simulink model "V40"  (R2017b)
settings: Solver=FixedStepAuto  StartTime=0.0  StopTime=50  FixedStep=dt  RelTol=1e-3
undefined symbols (not defined in the file): b_ref, c_bar, CG_ref_x, CG_ref_z, CL0, Clp, Clr, Cm0, Cmq, Cnp, Cnr, CX_d_ca_l, CX_d_ca_r, CX_d_ea_l, CX_d_ea_r, CX_d_r, d_ca_trim, D_CL_alpha, D_Cm_alpha, DCD_alpha, DCX_beta, dt, Earth, FW_P_RMAX_POS, FW_P_TC, FW_PR_FF, FW_PR_I, FW_PR_IMAX, FW_PR_P, FW_R_RMAX, FW_R_TC, FW_RR_FF, FW_RR_I, FW_RR_IMAX, FW_RR_P, FW_YR_FF, FW_YR_I, FW_YR_IMAX, FW_YR_P, g, h0, hgt_error_gain, hgt_gain_ff, K_L1, L1_ratio, lat0, lon0, mass0, max_climb_rate, max_sink_rate, min_sink_rate, Newton, p0, pitch0, Pitch_Kd, Pitch_Ki, pitch_sp_limit, pitch_time_constant, q0, r0 ... (+28)
libraries: simulink_extras x6, aerolibtransform2 x2, shared6dof x1, aerolibasang x1, simulink x1
(part 2 of 2)

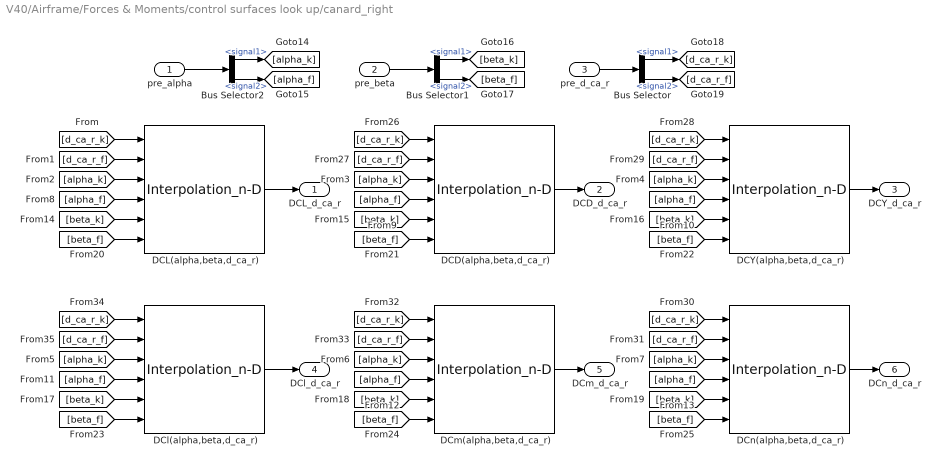
== system V40/Airframe/Forces & Moments/control surfaces look up/canard_right ==
  pre_alpha : Inport
  pre_beta : Inport  Port=2
  pre_d_ca_r : Inport  Port=3
  Bus Selector : BusSelector  OutputSignals=signal1,signal2
  Bus Selector1 : BusSelector  OutputSignals=signal1,signal2
  Bus Selector2 : BusSelector  OutputSignals=signal1,signal2
  DCD(alpha,beta,d_ca_r) : Interpolation_n-D  NumberOfTableDimensions=3  Table=CX_d_ca_r{2}  OutDataTypeStr=single
      settings: InputPortMap=u0,u1,u2,u3,u4,u5
  DCL(alpha,beta,d_ca_r) : Interpolation_n-D  NumberOfTableDimensions=3  Table=CX_d_ca_r{1}  OutDataTypeStr=single
      settings: InputPortMap=u0,u1,u2,u3,u4,u5
  DCY(alpha,beta,d_ca_r) : Interpolation_n-D  NumberOfTableDimensions=3  Table=CX_d_ca_r{4}  OutDataTypeStr=single
      settings: InputPortMap=u0,u1,u2,u3,u4,u5
  DCl(alpha,beta,d_ca_r) : Interpolation_n-D  NumberOfTableDimensions=3  Table=CX_d_ca_r{6}  OutDataTypeStr=single
      settings: InputPortMap=u0,u1,u2,u3,u4,u5
  DCm(alpha,beta,d_ca_r) : Interpolation_n-D  NumberOfTableDimensions=3  Table=CX_d_ca_r{3}  OutDataTypeStr=single
      settings: InputPortMap=u0,u1,u2,u3,u4,u5
  DCn(alpha,beta,d_ca_r) : Interpolation_n-D  NumberOfTableDimensions=3  Table=CX_d_ca_r{5}  OutDataTypeStr=single
      settings: InputPortMap=u0,u1,u2,u3,u4,u5
  DCL_d_ca_r : Outport
  DCD_d_ca_r : Outport  Port=2
  DCY_d_ca_r : Outport  Port=3
  DCl_d_ca_r : Outport  Port=4
  DCm_d_ca_r : Outport  Port=5
  DCn_d_ca_r : Outport  Port=6
  wires:
  Bus Selector1/2 -> [beta_f]  "<signal2>"
  DCY(alpha,beta,d_ca_r)/1 -> DCY_d_ca_r/1
  pre_beta/1 -> Bus Selector1/1
  Bus Selector/2 -> [d_ca_r_f]  "<signal2>"
  DCD(alpha,beta,d_ca_r)/1 -> DCD_d_ca_r/1
  DCl(alpha,beta,d_ca_r)/1 -> DCl_d_ca_r/1
  Bus Selector/1 -> [d_ca_r_k]  "<signal1>"
  Bus Selector2/1 -> [alpha_k]  "<signal1>"
  DCm(alpha,beta,d_ca_r)/1 -> DCm_d_ca_r/1
  Bus Selector2/2 -> [alpha_f]  "<signal2>"
  pre_alpha/1 -> Bus Selector2/1
  DCn(alpha,beta,d_ca_r)/1 -> DCn_d_ca_r/1
  DCL(alpha,beta,d_ca_r)/1 -> DCL_d_ca_r/1
  Bus Selector1/1 -> [beta_k]  "<signal1>"
  [d_ca_r_k] -> DCD(alpha,beta,d_ca_r)/1
  [beta_k] -> DCD(alpha,beta,d_ca_r)/5
  [d_ca_r_k] -> DCY(alpha,beta,d_ca_r)/1
  [beta_k] -> DCY(alpha,beta,d_ca_r)/5
  [alpha_k] -> DCY(alpha,beta,d_ca_r)/3
  [d_ca_r_k] -> DCn(alpha,beta,d_ca_r)/1
  [beta_k] -> DCn(alpha,beta,d_ca_r)/5
  [d_ca_r_k] -> DCm(alpha,beta,d_ca_r)/1
  [beta_k] -> DCm(alpha,beta,d_ca_r)/5
  [d_ca_r_k] -> DCL(alpha,beta,d_ca_r)/1
  [d_ca_r_f] -> DCL(alpha,beta,d_ca_r)/2
  [alpha_k] -> DCL(alpha,beta,d_ca_r)/3
  [alpha_f] -> DCL(alpha,beta,d_ca_r)/4
  [beta_k] -> DCL(alpha,beta,d_ca_r)/5
  [beta_f] -> DCL(alpha,beta,d_ca_r)/6
  [d_ca_r_f] -> DCD(alpha,beta,d_ca_r)/2
  [alpha_k] -> DCD(alpha,beta,d_ca_r)/3
  [alpha_f] -> DCD(alpha,beta,d_ca_r)/4
  [beta_f] -> DCD(alpha,beta,d_ca_r)/6
  [d_ca_r_f] -> DCY(alpha,beta,d_ca_r)/2
  [alpha_f] -> DCY(alpha,beta,d_ca_r)/4
  [beta_f] -> DCY(alpha,beta,d_ca_r)/6
  [d_ca_r_f] -> DCn(alpha,beta,d_ca_r)/2
  [alpha_k] -> DCn(alpha,beta,d_ca_r)/3
  [alpha_f] -> DCn(alpha,beta,d_ca_r)/4
  [beta_f] -> DCn(alpha,beta,d_ca_r)/6
  [d_ca_r_f] -> DCm(alpha,beta,d_ca_r)/2
  [alpha_k] -> DCm(alpha,beta,d_ca_r)/3
  [alpha_f] -> DCm(alpha,beta,d_ca_r)/4
  [beta_f] -> DCm(alpha,beta,d_ca_r)/6
  [d_ca_r_k] -> DCl(alpha,beta,d_ca_r)/1
  [d_ca_r_f] -> DCl(alpha,beta,d_ca_r)/2
  [alpha_k] -> DCl(alpha,beta,d_ca_r)/3
  [alpha_f] -> DCl(alpha,beta,d_ca_r)/4
  [beta_k] -> DCl(alpha,beta,d_ca_r)/5
  [beta_f] -> DCl(alpha,beta,d_ca_r)/6
  pre_d_ca_r/1 -> Bus Selector/1

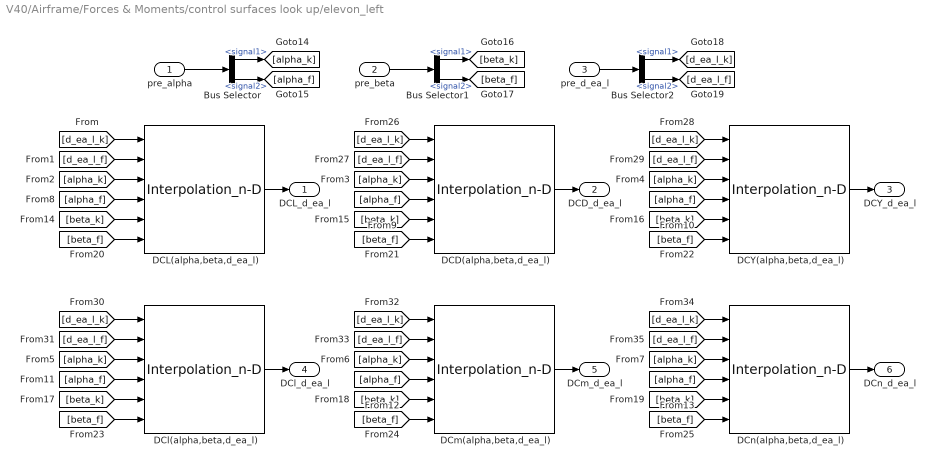
== system V40/Airframe/Forces & Moments/control surfaces look up/elevon_left  ==
  pre_alpha : Inport
  pre_beta : Inport  Port=2
  pre_d_ea_l : Inport  Port=3
  Bus Selector : BusSelector  OutputSignals=signal1,signal2
  Bus Selector1 : BusSelector  OutputSignals=signal1,signal2
  Bus Selector2 : BusSelector  OutputSignals=signal1,signal2
  DCD(alpha,beta,d_ea_l) : Interpolation_n-D  NumberOfTableDimensions=3  Table=CX_d_ea_l{2}  OutDataTypeStr=single
      settings: InputPortMap=u0,u1,u2,u3,u4,u5
  DCL(alpha,beta,d_ea_l) : Interpolation_n-D  NumberOfTableDimensions=3  Table=CX_d_ea_l{1}  OutDataTypeStr=single
      settings: InputPortMap=u0,u1,u2,u3,u4,u5
  DCY(alpha,beta,d_ea_l) : Interpolation_n-D  NumberOfTableDimensions=3  Table=CX_d_ea_l{4}  OutDataTypeStr=single
      settings: InputPortMap=u0,u1,u2,u3,u4,u5
  DCl(alpha,beta,d_ea_l) : Interpolation_n-D  NumberOfTableDimensions=3  Table=CX_d_ea_l{6}  OutDataTypeStr=single
      settings: InputPortMap=u0,u1,u2,u3,u4,u5
  DCm(alpha,beta,d_ea_l) : Interpolation_n-D  NumberOfTableDimensions=3  Table=CX_d_ea_l{3}  OutDataTypeStr=single
      settings: InputPortMap=u0,u1,u2,u3,u4,u5
  DCn(alpha,beta,d_ea_l) : Interpolation_n-D  NumberOfTableDimensions=3  Table=CX_d_ea_l{5}  OutDataTypeStr=single
      settings: InputPortMap=u0,u1,u2,u3,u4,u5
  DCL_d_ea_l : Outport
  DCD_d_ea_l : Outport  Port=2
  DCY_d_ea_l : Outport  Port=3
  DCl_d_ea_l : Outport  Port=4
  DCm_d_ea_l : Outport  Port=5
  DCn_d_ea_l : Outport  Port=6
  wires:
  Bus Selector1/2 -> [beta_f]  "<signal2>"
  DCY(alpha,beta,d_ea_l)/1 -> DCY_d_ea_l/1
  pre_beta/1 -> Bus Selector1/1
  Bus Selector2/2 -> [d_ea_l_f]  "<signal2>"
  DCD(alpha,beta,d_ea_l)/1 -> DCD_d_ea_l/1
  DCl(alpha,beta,d_ea_l)/1 -> DCl_d_ea_l/1
  Bus Selector2/1 -> [d_ea_l_k]  "<signal1>"
  Bus Selector/1 -> [alpha_k]  "<signal1>"
  DCm(alpha,beta,d_ea_l)/1 -> DCm_d_ea_l/1
  Bus Selector/2 -> [alpha_f]  "<signal2>"
  pre_alpha/1 -> Bus Selector/1
  DCn(alpha,beta,d_ea_l)/1 -> DCn_d_ea_l/1
  DCL(alpha,beta,d_ea_l)/1 -> DCL_d_ea_l/1
  Bus Selector1/1 -> [beta_k]  "<signal1>"
  [beta_k] -> DCL(alpha,beta,d_ea_l)/5
  [beta_f] -> DCL(alpha,beta,d_ea_l)/6
  [beta_k] -> DCD(alpha,beta,d_ea_l)/5
  [beta_f] -> DCD(alpha,beta,d_ea_l)/6
  [beta_k] -> DCY(alpha,beta,d_ea_l)/5
  [beta_f] -> DCY(alpha,beta,d_ea_l)/6
  [beta_k] -> DCl(alpha,beta,d_ea_l)/5
  [beta_f] -> DCl(alpha,beta,d_ea_l)/6
  [beta_k] -> DCm(alpha,beta,d_ea_l)/5
  [beta_f] -> DCm(alpha,beta,d_ea_l)/6
  [beta_k] -> DCn(alpha,beta,d_ea_l)/5
  [beta_f] -> DCn(alpha,beta,d_ea_l)/6
  [d_ea_l_k] -> DCD(alpha,beta,d_ea_l)/1
  [d_ea_l_k] -> DCY(alpha,beta,d_ea_l)/1
  [d_ea_l_k] -> DCn(alpha,beta,d_ea_l)/1
  [alpha_k] -> DCn(alpha,beta,d_ea_l)/3
  [d_ea_l_k] -> DCm(alpha,beta,d_ea_l)/1
  [alpha_k] -> DCm(alpha,beta,d_ea_l)/3
  [d_ea_l_k] -> DCl(alpha,beta,d_ea_l)/1
  [alpha_k] -> DCl(alpha,beta,d_ea_l)/3
  [d_ea_l_k] -> DCL(alpha,beta,d_ea_l)/1
  [d_ea_l_f] -> DCL(alpha,beta,d_ea_l)/2
  [alpha_k] -> DCL(alpha,beta,d_ea_l)/3
  [alpha_f] -> DCL(alpha,beta,d_ea_l)/4
  [d_ea_l_f] -> DCD(alpha,beta,d_ea_l)/2
  [alpha_k] -> DCD(alpha,beta,d_ea_l)/3
  [alpha_f] -> DCD(alpha,beta,d_ea_l)/4
  [d_ea_l_f] -> DCY(alpha,beta,d_ea_l)/2
  [alpha_k] -> DCY(alpha,beta,d_ea_l)/3
  [alpha_f] -> DCY(alpha,beta,d_ea_l)/4
  [d_ea_l_f] -> DCn(alpha,beta,d_ea_l)/2
  [alpha_f] -> DCn(alpha,beta,d_ea_l)/4
  [d_ea_l_f] -> DCm(alpha,beta,d_ea_l)/2
  [alpha_f] -> DCm(alpha,beta,d_ea_l)/4
  [d_ea_l_f] -> DCl(alpha,beta,d_ea_l)/2
  [alpha_f] -> DCl(alpha,beta,d_ea_l)/4
  pre_d_ea_l/1 -> Bus Selector2/1

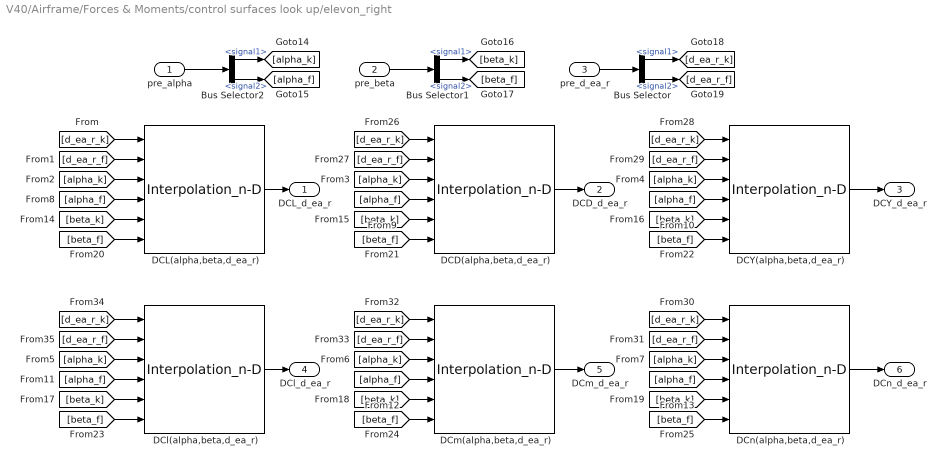
== system V40/Airframe/Forces & Moments/control surfaces look up/elevon_right  ==
  pre_alpha : Inport
  pre_beta : Inport  Port=2
  pre_d_ea_r : Inport  Port=3
  Bus Selector : BusSelector  OutputSignals=signal1,signal2
  Bus Selector1 : BusSelector  OutputSignals=signal1,signal2
  Bus Selector2 : BusSelector  OutputSignals=signal1,signal2
  DCD(alpha,beta,d_ea_r) : Interpolation_n-D  NumberOfTableDimensions=3  Table=CX_d_ea_r{2}  OutDataTypeStr=single
      settings: InputPortMap=u0,u1,u2,u3,u4,u5
  DCL(alpha,beta,d_ea_r) : Interpolation_n-D  NumberOfTableDimensions=3  Table=CX_d_ea_r{1}  OutDataTypeStr=single
      settings: InputPortMap=u0,u1,u2,u3,u4,u5
  DCY(alpha,beta,d_ea_r) : Interpolation_n-D  NumberOfTableDimensions=3  Table=CX_d_ea_r{4}  OutDataTypeStr=single
      settings: InputPortMap=u0,u1,u2,u3,u4,u5
  DCl(alpha,beta,d_ea_r) : Interpolation_n-D  NumberOfTableDimensions=3  Table=CX_d_ea_r{6}  OutDataTypeStr=single
      settings: InputPortMap=u0,u1,u2,u3,u4,u5
  DCm(alpha,beta,d_ea_r) : Interpolation_n-D  NumberOfTableDimensions=3  Table=CX_d_ea_r{3}  OutDataTypeStr=single
      settings: InputPortMap=u0,u1,u2,u3,u4,u5
  DCn(alpha,beta,d_ea_r) : Interpolation_n-D  NumberOfTableDimensions=3  Table=CX_d_ea_r{5}  OutDataTypeStr=single
      settings: InputPortMap=u0,u1,u2,u3,u4,u5
  DCL_d_ea_r : Outport
  DCD_d_ea_r : Outport  Port=2
  DCY_d_ea_r : Outport  Port=3
  DCl_d_ea_r : Outport  Port=4
  DCm_d_ea_r : Outport  Port=5
  DCn_d_ea_r : Outport  Port=6
  wires:
  Bus Selector1/2 -> [beta_f]  "<signal2>"
  DCY(alpha,beta,d_ea_r)/1 -> DCY_d_ea_r/1
  pre_beta/1 -> Bus Selector1/1
  Bus Selector/2 -> [d_ea_r_f]  "<signal2>"
  DCD(alpha,beta,d_ea_r)/1 -> DCD_d_ea_r/1
  DCl(alpha,beta,d_ea_r)/1 -> DCl_d_ea_r/1
  Bus Selector/1 -> [d_ea_r_k]  "<signal1>"
  Bus Selector2/1 -> [alpha_k]  "<signal1>"
  DCm(alpha,beta,d_ea_r)/1 -> DCm_d_ea_r/1
  Bus Selector2/2 -> [alpha_f]  "<signal2>"
  pre_alpha/1 -> Bus Selector2/1
  DCn(alpha,beta,d_ea_r)/1 -> DCn_d_ea_r/1
  DCL(alpha,beta,d_ea_r)/1 -> DCL_d_ea_r/1
  Bus Selector1/1 -> [beta_k]  "<signal1>"
  [beta_k] -> DCL(alpha,beta,d_ea_r)/5
  [beta_f] -> DCL(alpha,beta,d_ea_r)/6
  [beta_k] -> DCD(alpha,beta,d_ea_r)/5
  [beta_f] -> DCD(alpha,beta,d_ea_r)/6
  [beta_k] -> DCY(alpha,beta,d_ea_r)/5
  [beta_f] -> DCY(alpha,beta,d_ea_r)/6
  [beta_k] -> DCl(alpha,beta,d_ea_r)/5
  [beta_f] -> DCl(alpha,beta,d_ea_r)/6
  [beta_k] -> DCm(alpha,beta,d_ea_r)/5
  [beta_f] -> DCm(alpha,beta,d_ea_r)/6
  [beta_k] -> DCn(alpha,beta,d_ea_r)/5
  [beta_f] -> DCn(alpha,beta,d_ea_r)/6
  [d_ea_r_k] -> DCD(alpha,beta,d_ea_r)/1
  [d_ea_r_k] -> DCY(alpha,beta,d_ea_r)/1
  [d_ea_r_k] -> DCn(alpha,beta,d_ea_r)/1
  [d_ea_r_k] -> DCm(alpha,beta,d_ea_r)/1
  [d_ea_r_k] -> DCL(alpha,beta,d_ea_r)/1
  [d_ea_r_f] -> DCL(alpha,beta,d_ea_r)/2
  [alpha_k] -> DCL(alpha,beta,d_ea_r)/3
  [alpha_f] -> DCL(alpha,beta,d_ea_r)/4
  [d_ea_r_f] -> DCD(alpha,beta,d_ea_r)/2
  [alpha_k] -> DCD(alpha,beta,d_ea_r)/3
  [alpha_f] -> DCD(alpha,beta,d_ea_r)/4
  [d_ea_r_f] -> DCY(alpha,beta,d_ea_r)/2
  [alpha_k] -> DCY(alpha,beta,d_ea_r)/3
  [alpha_f] -> DCY(alpha,beta,d_ea_r)/4
  [d_ea_r_f] -> DCn(alpha,beta,d_ea_r)/2
  [alpha_k] -> DCn(alpha,beta,d_ea_r)/3
  [alpha_f] -> DCn(alpha,beta,d_ea_r)/4
  [d_ea_r_f] -> DCm(alpha,beta,d_ea_r)/2
  [alpha_k] -> DCm(alpha,beta,d_ea_r)/3
  [alpha_f] -> DCm(alpha,beta,d_ea_r)/4
  [d_ea_r_k] -> DCl(alpha,beta,d_ea_r)/1
  [d_ea_r_f] -> DCl(alpha,beta,d_ea_r)/2
  [alpha_k] -> DCl(alpha,beta,d_ea_r)/3
  [alpha_f] -> DCl(alpha,beta,d_ea_r)/4
  pre_d_ea_r/1 -> Bus Selector/1

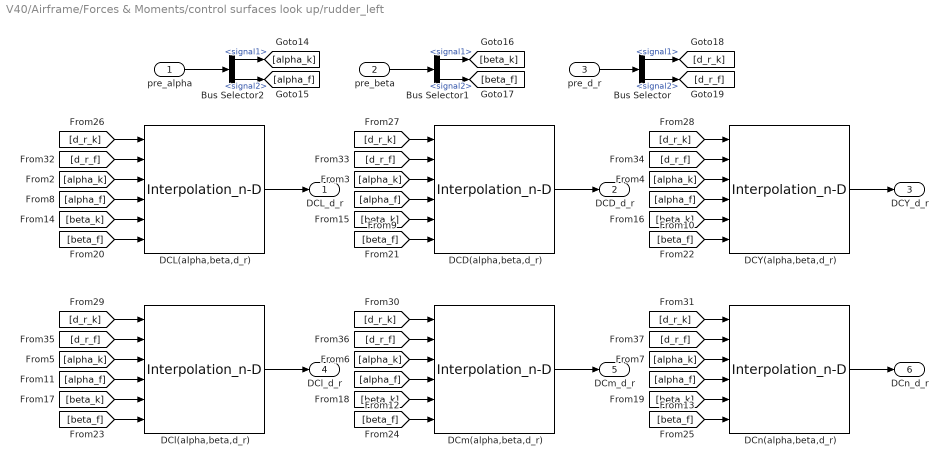
== system V40/Airframe/Forces & Moments/control surfaces look up/rudder_left ==
  pre_alpha : Inport
  pre_beta : Inport  Port=2
  pre_d_r : Inport  Port=3
  Bus Selector : BusSelector  OutputSignals=signal1,signal2
  Bus Selector1 : BusSelector  OutputSignals=signal1,signal2
  Bus Selector2 : BusSelector  OutputSignals=signal1,signal2
  DCD(alpha,beta,d_r) : Interpolation_n-D  NumberOfTableDimensions=3  Table=CX_d_r{2}  OutDataTypeStr=single
      settings: InputPortMap=u0,u1,u2,u3,u4,u5
  DCL(alpha,beta,d_r) : Interpolation_n-D  NumberOfTableDimensions=3  Table=CX_d_r{1}  OutDataTypeStr=single
      settings: InputPortMap=u0,u1,u2,u3,u4,u5
  DCY(alpha,beta,d_r) : Interpolation_n-D  NumberOfTableDimensions=3  Table=CX_d_r{4}  OutDataTypeStr=single
      settings: InputPortMap=u0,u1,u2,u3,u4,u5
  DCl(alpha,beta,d_r) : Interpolation_n-D  NumberOfTableDimensions=3  Table=CX_d_r{6}  OutDataTypeStr=single
      settings: InputPortMap=u0,u1,u2,u3,u4,u5
  DCm(alpha,beta,d_r) : Interpolation_n-D  NumberOfTableDimensions=3  Table=CX_d_r{3}  OutDataTypeStr=single
      settings: InputPortMap=u0,u1,u2,u3,u4,u5
  DCn(alpha,beta,d_r) : Interpolation_n-D  NumberOfTableDimensions=3  Table=CX_d_r{5}  OutDataTypeStr=single
      settings: InputPortMap=u0,u1,u2,u3,u4,u5
  DCL_d_r : Outport
  DCD_d_r : Outport  Port=2
  DCY_d_r : Outport  Port=3
  DCl_d_r : Outport  Port=4
  DCm_d_r : Outport  Port=5
  DCn_d_r : Outport  Port=6
  wires:
  Bus Selector1/2 -> [beta_f]  "<signal2>"
  DCY(alpha,beta,d_r)/1 -> DCY_d_r/1
  pre_beta/1 -> Bus Selector1/1
  Bus Selector/2 -> [d_r_f]  "<signal2>"
  DCD(alpha,beta,d_r)/1 -> DCD_d_r/1
  DCl(alpha,beta,d_r)/1 -> DCl_d_r/1
  Bus Selector/1 -> [d_r_k]  "<signal1>"
  Bus Selector2/1 -> [alpha_k]  "<signal1>"
  DCm(alpha,beta,d_r)/1 -> DCm_d_r/1
  Bus Selector2/2 -> [alpha_f]  "<signal2>"
  pre_alpha/1 -> Bus Selector2/1
  DCn(alpha,beta,d_r)/1 -> DCn_d_r/1
  DCL(alpha,beta,d_r)/1 -> DCL_d_r/1
  Bus Selector1/1 -> [beta_k]  "<signal1>"
  [d_r_k] -> DCD(alpha,beta,d_r)/1
  [beta_k] -> DCD(alpha,beta,d_r)/5
  [d_r_k] -> DCY(alpha,beta,d_r)/1
  [beta_k] -> DCY(alpha,beta,d_r)/5
  [alpha_k] -> DCY(alpha,beta,d_r)/3
  [d_r_k] -> DCn(alpha,beta,d_r)/1
  [beta_k] -> DCn(alpha,beta,d_r)/5
  [d_r_k] -> DCm(alpha,beta,d_r)/1
  [beta_k] -> DCm(alpha,beta,d_r)/5
  [d_r_k] -> DCL(alpha,beta,d_r)/1
  [d_r_f] -> DCL(alpha,beta,d_r)/2
  [alpha_k] -> DCL(alpha,beta,d_r)/3
  [alpha_f] -> DCL(alpha,beta,d_r)/4
  [beta_k] -> DCL(alpha,beta,d_r)/5
  [beta_f] -> DCL(alpha,beta,d_r)/6
  [d_r_f] -> DCD(alpha,beta,d_r)/2
  [alpha_k] -> DCD(alpha,beta,d_r)/3
  [alpha_f] -> DCD(alpha,beta,d_r)/4
  [beta_f] -> DCD(alpha,beta,d_r)/6
  [d_r_f] -> DCY(alpha,beta,d_r)/2
  [alpha_f] -> DCY(alpha,beta,d_r)/4
  [beta_f] -> DCY(alpha,beta,d_r)/6
  [d_r_f] -> DCn(alpha,beta,d_r)/2
  [alpha_k] -> DCn(alpha,beta,d_r)/3
  [alpha_f] -> DCn(alpha,beta,d_r)/4
  [beta_f] -> DCn(alpha,beta,d_r)/6
  [d_r_f] -> DCm(alpha,beta,d_r)/2
  [alpha_k] -> DCm(alpha,beta,d_r)/3
  [alpha_f] -> DCm(alpha,beta,d_r)/4
  [beta_f] -> DCm(alpha,beta,d_r)/6
  [d_r_k] -> DCl(alpha,beta,d_r)/1
  [d_r_f] -> DCl(alpha,beta,d_r)/2
  [alpha_k] -> DCl(alpha,beta,d_r)/3
  [alpha_f] -> DCl(alpha,beta,d_r)/4
  [beta_k] -> DCl(alpha,beta,d_r)/5
  [beta_f] -> DCl(alpha,beta,d_r)/6
  pre_d_r/1 -> Bus Selector/1

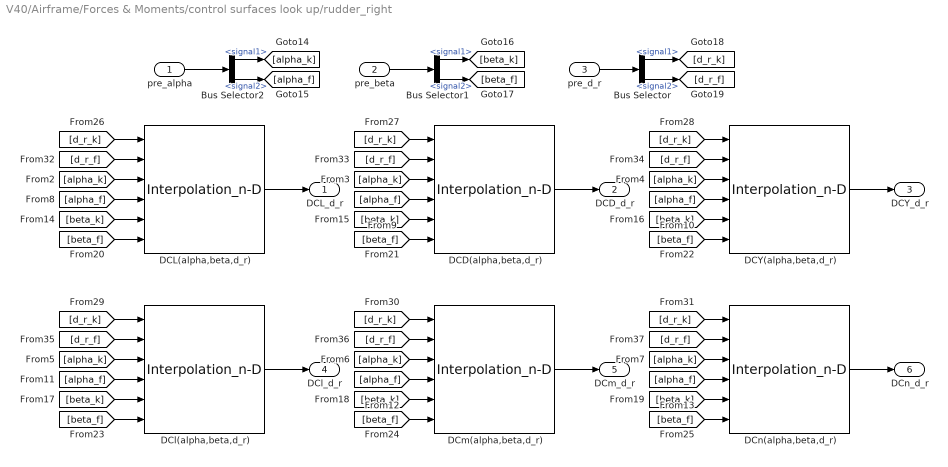
== system V40/Airframe/Forces & Moments/control surfaces look up/rudder_right ==
  pre_alpha : Inport
  pre_beta : Inport  Port=2
  pre_d_r : Inport  Port=3
  Bus Selector : BusSelector  OutputSignals=signal1,signal2
  Bus Selector1 : BusSelector  OutputSignals=signal1,signal2
  Bus Selector2 : BusSelector  OutputSignals=signal1,signal2
  DCD(alpha,beta,d_r) : Interpolation_n-D  NumberOfTableDimensions=3  Table=CX_d_r{2}  OutDataTypeStr=single
      settings: InputPortMap=u0,u1,u2,u3,u4,u5
  DCL(alpha,beta,d_r) : Interpolation_n-D  NumberOfTableDimensions=3  Table=CX_d_r{1}  OutDataTypeStr=single
      settings: InputPortMap=u0,u1,u2,u3,u4,u5
  DCY(alpha,beta,d_r) : Interpolation_n-D  NumberOfTableDimensions=3  Table=CX_d_r{4}  OutDataTypeStr=single
      settings: InputPortMap=u0,u1,u2,u3,u4,u5
  DCl(alpha,beta,d_r) : Interpolation_n-D  NumberOfTableDimensions=3  Table=CX_d_r{6}  OutDataTypeStr=single
      settings: InputPortMap=u0,u1,u2,u3,u4,u5
  DCm(alpha,beta,d_r) : Interpolation_n-D  NumberOfTableDimensions=3  Table=CX_d_r{3}  OutDataTypeStr=single
      settings: InputPortMap=u0,u1,u2,u3,u4,u5
  DCn(alpha,beta,d_r) : Interpolation_n-D  NumberOfTableDimensions=3  Table=CX_d_r{5}  OutDataTypeStr=single
      settings: InputPortMap=u0,u1,u2,u3,u4,u5
  DCL_d_r : Outport
  DCD_d_r : Outport  Port=2
  DCY_d_r : Outport  Port=3
  DCl_d_r : Outport  Port=4
  DCm_d_r : Outport  Port=5
  DCn_d_r : Outport  Port=6
  wires:
  Bus Selector1/2 -> [beta_f]  "<signal2>"
  DCY(alpha,beta,d_r)/1 -> DCY_d_r/1
  pre_beta/1 -> Bus Selector1/1
  Bus Selector/2 -> [d_r_f]  "<signal2>"
  DCD(alpha,beta,d_r)/1 -> DCD_d_r/1
  DCl(alpha,beta,d_r)/1 -> DCl_d_r/1
  Bus Selector/1 -> [d_r_k]  "<signal1>"
  Bus Selector2/1 -> [alpha_k]  "<signal1>"
  DCm(alpha,beta,d_r)/1 -> DCm_d_r/1
  Bus Selector2/2 -> [alpha_f]  "<signal2>"
  pre_alpha/1 -> Bus Selector2/1
  DCn(alpha,beta,d_r)/1 -> DCn_d_r/1
  DCL(alpha,beta,d_r)/1 -> DCL_d_r/1
  Bus Selector1/1 -> [beta_k]  "<signal1>"
  [d_r_k] -> DCD(alpha,beta,d_r)/1
  [beta_k] -> DCD(alpha,beta,d_r)/5
  [d_r_k] -> DCY(alpha,beta,d_r)/1
  [beta_k] -> DCY(alpha,beta,d_r)/5
  [alpha_k] -> DCY(alpha,beta,d_r)/3
  [d_r_k] -> DCn(alpha,beta,d_r)/1
  [beta_k] -> DCn(alpha,beta,d_r)/5
  [d_r_k] -> DCm(alpha,beta,d_r)/1
  [beta_k] -> DCm(alpha,beta,d_r)/5
  [d_r_k] -> DCL(alpha,beta,d_r)/1
  [d_r_f] -> DCL(alpha,beta,d_r)/2
  [alpha_k] -> DCL(alpha,beta,d_r)/3
  [alpha_f] -> DCL(alpha,beta,d_r)/4
  [beta_k] -> DCL(alpha,beta,d_r)/5
  [beta_f] -> DCL(alpha,beta,d_r)/6
  [d_r_f] -> DCD(alpha,beta,d_r)/2
  [alpha_k] -> DCD(alpha,beta,d_r)/3
  [alpha_f] -> DCD(alpha,beta,d_r)/4
  [beta_f] -> DCD(alpha,beta,d_r)/6
  [d_r_f] -> DCY(alpha,beta,d_r)/2
  [alpha_f] -> DCY(alpha,beta,d_r)/4
  [beta_f] -> DCY(alpha,beta,d_r)/6
  [d_r_f] -> DCn(alpha,beta,d_r)/2
  [alpha_k] -> DCn(alpha,beta,d_r)/3
  [alpha_f] -> DCn(alpha,beta,d_r)/4
  [beta_f] -> DCn(alpha,beta,d_r)/6
  [d_r_f] -> DCm(alpha,beta,d_r)/2
  [alpha_k] -> DCm(alpha,beta,d_r)/3
  [alpha_f] -> DCm(alpha,beta,d_r)/4
  [beta_f] -> DCm(alpha,beta,d_r)/6
  [d_r_k] -> DCl(alpha,beta,d_r)/1
  [d_r_f] -> DCl(alpha,beta,d_r)/2
  [alpha_k] -> DCl(alpha,beta,d_r)/3
  [alpha_f] -> DCl(alpha,beta,d_r)/4
  [beta_k] -> DCl(alpha,beta,d_r)/5
  [beta_f] -> DCl(alpha,beta,d_r)/6
  pre_d_r/1 -> Bus Selector/1

== system V40/Airframe/Forces & Moments/summation/coef computation ==
  In : Inport
  Add1 : Sum  Inputs=+++++++++
  Demux : Demux  Outputs=9
  Out : Outport
  wires:
  In/1 -> Demux/1
  Add1/1 -> Out/1
  Demux/1 -> Add1/1
  Demux/9 -> Add1/9
  Demux/8 -> Add1/8
  Demux/7 -> Add1/7
  Demux/6 -> Add1/6
  Demux/5 -> Add1/5
  Demux/4 -> Add1/4
  Demux/2 -> Add1/2
  Demux/3 -> Add1/3

== system V40/Airframe/Forces & Moments/summation/coef computation1 ==
  In : Inport
  Add1 : Sum  Inputs=++++++++
  Demux : Demux  Outputs=8
  Out : Outport
  wires:
  In/1 -> Demux/1
  Add1/1 -> Out/1
  Demux/1 -> Add1/1
  Demux/2 -> Add1/2
  Demux/3 -> Add1/3
  Demux/4 -> Add1/4
  Demux/5 -> Add1/5
  Demux/6 -> Add1/6
  Demux/7 -> Add1/7
  Demux/8 -> Add1/8

== system V40/Airframe/Forces & Moments/summation/coef computation2 ==
  In : Inport
  Add1 : Sum  Inputs=+++++++
  Demux : Demux  Outputs=7
  Out : Outport
  wires:
  In/1 -> Demux/1
  Add1/1 -> Out/1
  Demux/1 -> Add1/1
  Demux/2 -> Add1/2
  Demux/3 -> Add1/3
  Demux/4 -> Add1/4
  Demux/5 -> Add1/5
  Demux/6 -> Add1/6
  Demux/7 -> Add1/7

== system V40/Airframe/Forces & Moments/summation/coef computation3 ==
  In : Inport
  Add1 : Sum  Inputs=++++++++
  Demux : Demux  Outputs=8
  Out : Outport
  wires:
  In/1 -> Demux/1
  Add1/1 -> Out/1
  Demux/7 -> Add1/7
  Demux/1 -> Add1/1
  Demux/2 -> Add1/2
  Demux/3 -> Add1/3
  Demux/4 -> Add1/4
  Demux/5 -> Add1/5
  Demux/6 -> Add1/6
  Demux/8 -> Add1/8

== system V40/Airframe/Forces & Moments/summation/coef computation4 ==
  In : Inport
  Add1 : Sum  Inputs=++++++++++
  Demux : Demux  Outputs=10
  Out : Outport
  wires:
  Add1/1 -> Out/1
  In/1 -> Demux/1
  Demux/1 -> Add1/1
  Demux/2 -> Add1/2
  Demux/3 -> Add1/3
  Demux/4 -> Add1/4
  Demux/5 -> Add1/5
  Demux/6 -> Add1/6
  Demux/7 -> Add1/7
  Demux/8 -> Add1/8
  Demux/9 -> Add1/9
  Demux/10 -> Add1/10

== system V40/Airframe/Forces & Moments/summation/coef computation5 ==
  In : Inport
  Add1 : Sum  Inputs=++++++++
  Demux : Demux  Outputs=8
  Out : Outport
  wires:
  Add1/1 -> Out/1
  In/1 -> Demux/1
  Demux/1 -> Add1/1
  Demux/2 -> Add1/2
  Demux/3 -> Add1/3
  Demux/4 -> Add1/4
  Demux/5 -> Add1/5
  Demux/6 -> Add1/6
  Demux/7 -> Add1/7
  Demux/8 -> Add1/8

== system V40/FLY_CTRL_SYS/ATT_CTRL(PID)/U_SURF/pitch_rate_ctrl ==
  pitch_rate_sp : Inport
  pitch_rate_est : Inport  Port=2
  FW_PR_FF : Gain  Gain=FW_PR_FF
  FW_PR_I : Gain  Gain=FW_PR_I
  FW_PR_P : Gain  Gain=FW_PR_P
  Integrator Limited1 : Integrator  LimitOutput=on  UpperSaturationLimit=FW_PR_IMAX  LowerSaturationLimit=-FW_PR_IMAX
  Saturation3 : Saturate  UpperLimit=1  LowerLimit=-1
  Sum4 : Sum  Inputs=|+-
  Sum5 : Sum  Inputs=+++
  u_pitch : Outport
  wires:
  Saturation3/1 -> u_pitch/1
  FW_PR_FF/1 -> Sum5/1
  pitch_rate_est/1 -> Sum4/2
  Sum5/1 -> Saturation3/1
  pitch_rate_sp/1 -> Sum4/1, FW_PR_FF/1
  FW_PR_P/1 -> Sum5/2
  Sum4/1 -> FW_PR_I/1, FW_PR_P/1
  Integrator Limited1/1 -> Sum5/3
  FW_PR_I/1 -> Integrator Limited1/1

== system V40/FLY_CTRL_SYS/ATT_CTRL(PID)/U_SURF/roll_rate_ctrl ==
  roll_rate_sp : Inport
  roll_rate_est : Inport  Port=2
  FW_RR_FF : Gain  Gain=FW_RR_FF
  FW_RR_I : Gain  Gain=FW_RR_I
  FW_RR_P : Gain  Gain=FW_RR_P
  Integrator Limited1 : Integrator  LimitOutput=on  UpperSaturationLimit=FW_RR_IMAX  LowerSaturationLimit=-FW_RR_IMAX
  Saturation3 : Saturate  UpperLimit=1  LowerLimit=-1
  Sum4 : Sum  Inputs=|+-
  Sum5 : Sum  Inputs=+++
  u_roll : Outport
  wires:
  Saturation3/1 -> u_roll/1
  FW_RR_FF/1 -> Sum5/1
  roll_rate_est/1 -> Sum4/2
  Sum5/1 -> Saturation3/1
  roll_rate_sp/1 -> Sum4/1, FW_RR_FF/1
  FW_RR_P/1 -> Sum5/2
  Sum4/1 -> FW_RR_P/1, FW_RR_I/1
  Integrator Limited1/1 -> Sum5/3
  FW_RR_I/1 -> Integrator Limited1/1

== system V40/FLY_CTRL_SYS/ATT_CTRL(PID)/U_SURF/yaw_rate_ctrl ==
  yaw_rate_sp : Inport
  yaw_rate_est : Inport  Port=2
  FW_YR_FF : Gain  Gain=FW_YR_FF
  FW_YR_I : Gain  Gain=FW_YR_I
  FW_YR_P : Gain  Gain=FW_YR_P
  Integrator Limited1 : Integrator  LimitOutput=on  UpperSaturationLimit=FW_YR_IMAX  LowerSaturationLimit=-FW_YR_IMAX
  Saturation3 : Saturate  UpperLimit=1  LowerLimit=-1
  Sum4 : Sum  Inputs=|+-
  Sum5 : Sum  Inputs=+++
  u_yaw : Outport
  wires:
  Saturation3/1 -> u_yaw/1
  FW_YR_FF/1 -> Sum5/1
  yaw_rate_est/1 -> Sum4/2
  Sum5/1 -> Saturation3/1
  yaw_rate_sp/1 -> Sum4/1, FW_YR_FF/1
  FW_YR_P/1 -> Sum5/2
  Sum4/1 -> FW_YR_I/1, FW_YR_P/1
  Integrator Limited1/1 -> Sum5/3
  FW_YR_I/1 -> Integrator Limited1/1

== system V40/FLY_CTRL_SYS/Guidance_Law/L1/Switch Case Action Subsystem ==
  vec_A2plane_UNIT : Inport
  ground_v_2d : Inport  Port=2
  Action Port : ActionPort  ActionType=case
  Demux : Demux  Outputs=2
  Dot Product1 : DotProduct  InputSameDT=on  OutDataTypeStr=Inherit: Inherit via internal rule
  Gain : Gain  Gain=-1
  MATLAB Function5 : MATLAB Function  TreatAsAtomicUnit=on
  Trigonometric Function : Trigonometry  Operator=atan2
  Trigonometric Function1 : Trigonometry  Operator=atan2
  eta : Outport
  nav_bearing : Outport  Port=2
  wires:
  vec_A2plane_UNIT/1 -> Gain/1
  ground_v_2d/1 -> Dot Product1/1, MATLAB Function5/1(vec1)
  Gain/1 -> Demux/1, Dot Product1/2, MATLAB Function5/2(vec2)
  MATLAB Function5/1(vec_mol) -> Trigonometric Function/1
  Dot Product1/1 -> Trigonometric Function/2
  Trigonometric Function/1 -> eta/1
  Demux/2 -> Trigonometric Function1/1
  Demux/1 -> Trigonometric Function1/2
  Trigonometric Function1/1 -> nav_bearing/1

== system V40/FLY_CTRL_SYS/Guidance_Law/L1/Switch Case Action Subsystem1 ==
  vec_B2plane_UNIT : Inport
  ground_v_2d : Inport  Port=2
  Action Port : ActionPort  ActionType=case
  Demux : Demux  Outputs=2
  Dot Product1 : DotProduct  InputSameDT=on  OutDataTypeStr=Inherit: Inherit via internal rule
  Gain : Gain  Gain=-1
  MATLAB Function5 : MATLAB Function  TreatAsAtomicUnit=on
  Trigonometric Function : Trigonometry  Operator=atan2
  Trigonometric Function1 : Trigonometry  Operator=atan2
  eta : Outport
  nav_bearing : Outport  Port=2
  wires:
  vec_B2plane_UNIT/1 -> Gain/1
  Gain/1 -> Demux/1, Dot Product1/2, MATLAB Function5/2(vec2)
  Trigonometric Function1/1 -> nav_bearing/1
  Demux/2 -> Trigonometric Function1/1
  Demux/1 -> Trigonometric Function1/2
  Dot Product1/1 -> Trigonometric Function/2
  Trigonometric Function/1 -> eta/1
  MATLAB Function5/1(vec_mol) -> Trigonometric Function/1
  ground_v_2d/1 -> MATLAB Function5/1(vec1), Dot Product1/1

== system V40/FLY_CTRL_SYS/Guidance_Law/L1/Switch Case Action Subsystem2 ==
  vec_AB_UNIT : Inport
  vec_A2plane : Inport  Port=2
  ground_v_2d : Inport  Port=3
  L1_distance : Inport  Port=4
  Action Port : ActionPort  ActionType=case
  Add : Sum
  Add1 : Sum
  Constant : Constant  Value=0.1
  Demux : Demux  Outputs=2
  Divide : Product  Inputs=*/
  Dot Product1 : DotProduct  InputSameDT=on  OutDataTypeStr=Inherit: Inherit via internal rule
  MATLAB Function1 : MATLAB Function  TreatAsAtomicUnit=on
  MATLAB Function5 : MATLAB Function  TreatAsAtomicUnit=on
  Saturation : Saturate  UpperLimit=0.7071  LowerLimit=-0.7071
  Switch : Switch  Criteria=u2 > Threshold  Threshold=0.1
  Trigonometric Function : Trigonometry  Operator=atan2
  Trigonometric Function1 : Trigonometry  Operator=asin
  Trigonometric Function2 : Trigonometry  Operator=atan2
  eta : Outport
  nav_bearing : Outport  Port=2
  wires:
  vec_AB_UNIT/1 -> Demux/1, MATLAB Function1/2(vec2), Dot Product1/2, MATLAB Function5/2(vec2)
  ground_v_2d/1 -> MATLAB Function5/1(vec1), Dot Product1/1
  MATLAB Function5/1(vec_mol) -> Trigonometric Function/1
  Dot Product1/1 -> Trigonometric Function/2
  Trigonometric Function/1 -> Add/1  "eta2"
  vec_A2plane/1 -> MATLAB Function1/1(vec1)
  MATLAB Function1/1(vec_mol) -> Divide/1
  L1_distance/1 -> Switch/2, Switch/1
  Constant/1 -> Switch/3
  Switch/1 -> Divide/2
  Divide/1 -> Saturation/1
  Saturation/1 -> Trigonometric Function1/1
  Trigonometric Function1/1 -> Add/2, Add1/1  "eta1"
  Add/1 -> eta/1
  Demux/1 -> Trigonometric Function2/2
  Demux/2 -> Trigonometric Function2/1
  Trigonometric Function2/1 -> Add1/2
  Add1/1 -> nav_bearing/1

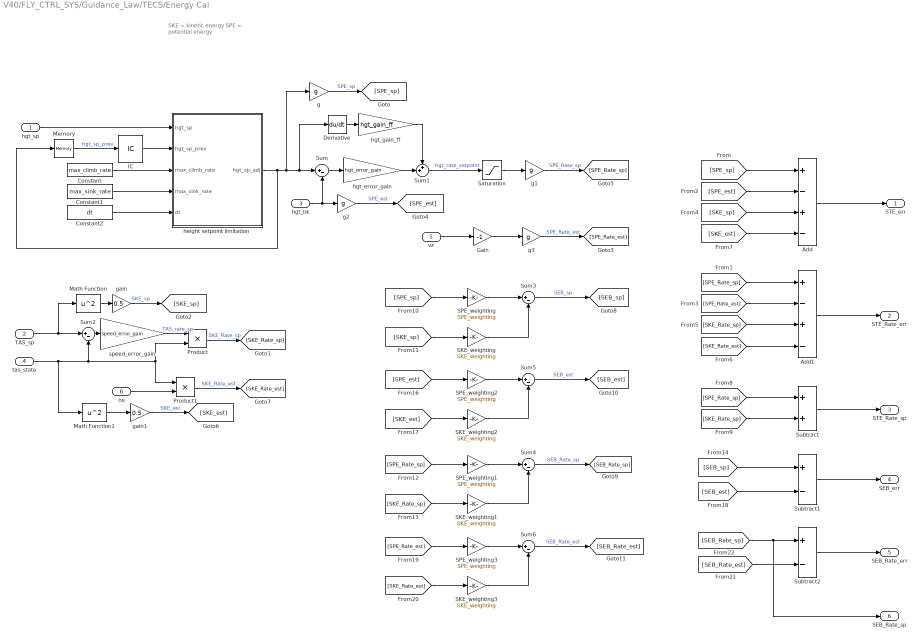
== system V40/FLY_CTRL_SYS/Guidance_Law/TECS/Energy Cal ==
  note: SKE = kinetic energy
      | SPE = potential energy
  hgt_sp : Inport
  TAS_sp : Inport  Port=2
  hgt_bk : Inport  Port=3
  tas_state : Inport  Port=4
  vz : Inport  Port=5
  nx : Inport  Port=6
  Add : Sum  Inputs=+-+-
  Add1 : Sum  Inputs=+-+-
  Constant : Constant  Value=max_climb_rate
  Constant1 : Constant  Value=max_sink_rate
  Constant2 : Constant  Value=dt
  Derivative : Derivative
  Gain : Gain  Gain=-1
  IC : InitialCondition  Value=-z0
  Math Function : Math  Operator=square  SaturateOnIntegerOverflow=on
  Math Function1 : Math  Operator=square  SaturateOnIntegerOverflow=on
  Memory : Memory
  Product : Product
  Product1 : Product
  SKE_weighting{,1..3} (4 alike) : Gain  Gain=SKE_weighting
  SPE_weighting{,1..3} (4 alike) : Gain  Gain=SPE_weighting
  Saturation : Saturate  UpperLimit=max_climb_rate  LowerLimit=-min_sink_rate
  Subtract : Sum
  Subtract1 : Sum  Inputs=+-
  Subtract2 : Sum  Inputs=+-
  Sum{,2..6} (6 alike) : Sum  Inputs=|+-
  Sum1 : Sum  Inputs=++|
  g{,1..3} (4 alike) : Gain  Gain=g
  gain : Gain  Gain=0.5
  gain1 : Gain  Gain=0.5
  height setpoint limitation : MATLAB Function  TreatAsAtomicUnit=on
  hgt_error_gain : Gain  Gain=hgt_error_gain
  hgt_gain_ff : Gain  Gain=hgt_gain_ff
  speed_error_gain : Gain  Gain=speed_error_gain
  STE_err : Outport
  STE_Rate_err : Outport  Port=2
  STE_Rate_sp : Outport  Port=3
  SEB_err : Outport  Port=4
  SEB_Rate_err : Outport  Port=5
  SEB_Rate_sp : Outport  Port=6
  wires:
  [SKE_est] -> Add/4
  vz/1 -> Gain/1
  Add1/1 -> STE_Rate_err/1
  hgt_error_gain/1 -> Sum1/2
  [SKE_Rate_est] -> Add1/4
  g1/1 -> [SPE_Rate_sp]  "SPE_Rate_sp"
  Derivative/1 -> hgt_gain_ff/1
  g/1 -> [SPE_sp]  "SPE_sp"
  Product1/1 -> [SKE_Rate_est]  "SKE_Rate_est"
  speed_error_gain/1 -> Product/1  "TAS_rate_sp"
  g2/1 -> [SPE_est]  "SPE_est"
  g3/1 -> [SPE_Rate_est]  "SPE_Rate_est"
  Sum/1 -> hgt_error_gain/1
  gain/1 -> [SKE_sp]  "SKE_sp"
  Math Function1/1 -> gain1/1
  [SPE_Rate_sp] -> Add1/1
  hgt_gain_ff/1 -> Sum1/1
  Math Function/1 -> gain/1
  gain1/1 -> [SKE_est]  "SKE_est"
  Product/1 -> [SKE_Rate_sp]  "SKE_Rate_sp"
  nx/1 -> Product1/2
  [SKE_Rate_sp] -> Add1/3
  [SKE_sp] -> Add/3
  Gain/1 -> g3/1
  Sum2/1 -> speed_error_gain/1
  Sum1/1 -> Saturation/1  "hgt_rate_setpoint"
  [SPE_est] -> Add/2
  [SPE_Rate_est] -> Add1/2
  hgt_bk/1 -> Sum/2, g2/1
  tas_state/1 -> Sum2/2, Product/2, Product1/1, Math Function1/1
  TAS_sp/1 -> Math Function/1, Sum2/1
  Add/1 -> STE_err/1
  [SPE_sp] -> Add/1
  [SPE_Rate_sp] -> Subtract/1
  [SKE_Rate_sp] -> Subtract/2
  Subtract/1 -> STE_Rate_sp/1
  [SPE_sp] -> SPE_weighting/1
  SPE_weighting/1 -> Sum3/1
  [SKE_sp] -> SKE_weighting/1
  SKE_weighting/1 -> Sum3/2
  Sum3/1 -> [SEB_sp]  "SEB_sp"
  [SKE_Rate_sp] -> SKE_weighting1/1
  SKE_weighting1/1 -> Sum4/2
  [SPE_Rate_sp] -> SPE_weighting1/1
  Sum4/1 -> [SEB_Rate_sp]  "SEB_Rate_sp"
  SPE_weighting1/1 -> Sum4/1
  [SKE_est] -> SKE_weighting2/1
  SKE_weighting2/1 -> Sum5/2
  [SPE_est] -> SPE_weighting2/1
  SPE_weighting2/1 -> Sum5/1
  Sum5/1 -> [SEB_est]  "SEB_est"
  SKE_weighting3/1 -> Sum6/2
  [SPE_Rate_est] -> SPE_weighting3/1
  SPE_weighting3/1 -> Sum6/1
  [SKE_Rate_est] -> SKE_weighting3/1
  Sum6/1 -> [SEB_Rate_est]  "SEB_Rate_est"
  [SEB_sp] -> Subtract1/1
  [SEB_est] -> Subtract1/2
  Subtract1/1 -> SEB_err/1
  [SEB_Rate_sp] -> SEB_Rate_sp/1, Subtract2/1
  [SEB_Rate_est] -> Subtract2/2
  Subtract2/1 -> SEB_Rate_err/1
  height setpoint limitation/1(hgt_sp_adj) -> Sum/1, Derivative/1, g/1, Memory/1
  Saturation/1 -> g1/1
  Constant/1 -> height setpoint limitation/3(max_climb_rate)
  Constant2/1 -> height setpoint limitation/5(dt)
  Constant1/1 -> height setpoint limitation/4(max_sink_rate)
  Memory/1 -> IC/1  "hgt_sp_prev"
  IC/1 -> height setpoint limitation/2(hgt_sp_prev)
  hgt_sp/1 -> height setpoint limitation/1(hgt_sp)

== matlab function V40/FLY_CTRL_SYS/ATT_CTRL(PID)/euler_rate_sp/yaw rate for coordinated flight ==
  data: euler input; yaw_rate_sp output; Vb input; g input
function yaw_rate_sp = fcn(euler, Vb, g)

yaw_rate_sp = g * tan(euler(1)) * cos(euler(2)) / abs(Vb(1));

== matlab function V40/FLY_CTRL_SYS/ATT_CTRL(PID)/euler_rate_sp/Euler_err to Euler_Rate ==
  data: euler_err input; euler_rate_sp output; euler_angle input
function euler_rate_sp = fcn(euler_err, euler_angle)
roll = euler_angle(1);
pitch = euler_angle(2);

euler_rate_sp = [1   0           -sin(pitch);
            0   cos(roll)    sin(roll)*cos(pitch);
            0   -sin(roll)   cos(roll)*cos(pitch)] * reshape(euler_err,3,1);

== matlab function V40/FLY_CTRL_SYS/Guidance_Law/L1/MATLAB Function ==
  data: PointA input; Vec output; PointB input
function Vec   = LB2VEC(PointA, PointB)
R2D = 180.0/pi;
D2R = 1.0/R2D;
RADIUS_OF_EARTH = 6371000;
% Vec1 = (PointB(1)-PointA(1))*D2R*RADIUS_OF_EARTH;
% Vec2 = (PointB(2)-PointA(2))*cosd(PointA(1))*D2R*RADIUS_OF_EARTH;
Vec = [(PointB(1)-PointA(1))*D2R*RADIUS_OF_EARTH,(PointB(2)-PointA(2))*cosd(PointA(1))*D2R*RADIUS_OF_EARTH];

== matlab function V40/FLY_CTRL_SYS/Guidance_Law/L1/MATLAB Function1 ==
  data: PointA input; Vec output; PointB input
function Vec   = LB2VEC(PointA, PointB)
R2D = 180.0/pi;
D2R = 1.0/R2D;
RADIUS_OF_EARTH = 6371000;
% Vec1 = (PointB(1)-PointA(1))*D2R*RADIUS_OF_EARTH;
% Vec2 = (PointB(2)-PointA(2))*cosd(PointA(1))*D2R*RADIUS_OF_EARTH;
Vec = [(PointB(1)-PointA(1))*D2R*RADIUS_OF_EARTH,(PointB(2)-PointA(2))*cosd(PointA(1))*D2R*RADIUS_OF_EARTH];

== matlab function V40/FLY_CTRL_SYS/Guidance_Law/L1/MATLAB Function2 ==
  data: vec1 input; vec_mol output; vec2 input
function vec_mol = Vec_CrossProduct2d(vec1,vec2)
vec_mol = vec1(1)*vec2(2)-vec1(2)*vec2(1);

== matlab function V40/FLY_CTRL_SYS/Guidance_Law/L1/MATLAB Function3 ==
  data: PointA input; Vec output; PointB input
function Vec   = LB2VEC(PointA, PointB)
R2D = 180.0/pi;
D2R = 1.0/R2D;
RADIUS_OF_EARTH = 6371000;
% Vec1 = (PointB(1)-PointA(1))*D2R*RADIUS_OF_EARTH;
% Vec2 = (PointB(2)-PointA(2))*cosd(PointA(1))*D2R*RADIUS_OF_EARTH;
Vec = [(PointB(1)-PointA(1))*D2R*RADIUS_OF_EARTH,(PointB(2)-PointA(2))*cosd(PointA(1))*D2R*RADIUS_OF_EARTH];

== matlab function V40/FLY_CTRL_SYS/Guidance_Law/L1/MATLAB Function4 ==
  data: PointA input; Vec output; PointB input
function Vec   = LB2VEC(PointA, PointB)
R2D = 180.0/pi;
D2R = 1.0/R2D;
RADIUS_OF_EARTH = 6371000;
% Vec1 = (PointB(1)-PointA(1))*D2R*RADIUS_OF_EARTH;
% Vec2 = (PointB(2)-PointA(2))*cosd(PointA(1))*D2R*RADIUS_OF_EARTH;
Vec = [(PointB(1)-PointA(1))*D2R*RADIUS_OF_EARTH,(PointB(2)-PointA(2))*cosd(PointA(1))*D2R*RADIUS_OF_EARTH];

== matlab function V40/FLY_CTRL_SYS/Guidance_Law/L1/MATLAB Function5 ==
  data: vec1 input; vec_mol output; vec2 input
function vec_mol = Vec_CrossProduct2d(vec1,vec2)
vec_mol = vec1(1)*vec2(2)-vec1(2)*vec2(1);

== matlab function V40/FLY_CTRL_SYS/Guidance_Law/L1/MATLAB Function6 ==
  data: disA2P input; LogicCase output; L1_dis input; alongTrackDis input; AB2BP_bearing input; V2AB_bearing input
function LogicCase = fcn(disA2P,L1_dis,alongTrackDis,AB2BP_bearing,V2AB_bearing)
R2D = 180.0/pi;
D2R = 1.0/R2D;

if(disA2P > 1.0)
    disA2P_max = disA2P;
else
    disA2P_max = 1.0;
end

if((disA2P > L1_dis) && (alongTrackDis/disA2P_max < -0.7071))
    LogicCase = 1;
elseif((abs(AB2BP_bearing)< 100.0*D2R) || (abs(V2AB_bearing)>=90.0*D2R))
    LogicCase = 2;
else
    LogicCase = 3;
end

== matlab function V40/FLY_CTRL_SYS/Guidance_Law/L1/Switch Case Action Subsystem/MATLAB Function5 ==
  data: vec1 input; vec_mol output; vec2 input
function vec_mol = Vec_CrossProduct2d(vec1,vec2)
vec_mol = vec1(1)*vec2(2)-vec1(2)*vec2(1);

== matlab function V40/FLY_CTRL_SYS/Guidance_Law/L1/Switch Case Action Subsystem1/MATLAB Function5 ==
  data: vec1 input; vec_mol output; vec2 input
function vec_mol = Vec_CrossProduct2d(vec1,vec2)
vec_mol = vec1(1)*vec2(2)-vec1(2)*vec2(1);

== matlab function V40/FLY_CTRL_SYS/Guidance_Law/L1/Switch Case Action Subsystem2/MATLAB Function1 ==
  data: vec1 input; vec_mol output; vec2 input
function vec_mol = Vec_CrossProduct2d(vec1,vec2)
vec_mol = vec1(1)*vec2(2)-vec1(2)*vec2(1);

== matlab function V40/FLY_CTRL_SYS/Guidance_Law/L1/Switch Case Action Subsystem2/MATLAB Function5 ==
  data: vec1 input; vec_mol output; vec2 input
function vec_mol = Vec_CrossProduct2d(vec1,vec2)
vec_mol = vec1(1)*vec2(2)-vec1(2)*vec2(1);

== matlab function V40/FLY_CTRL_SYS/Guidance_Law/TECS/Energy Cal/height setpoint limitation ==
  data: hgt_sp input; hgt_sp_adj output; hgt_sp_prev input; max_climb_rate input; max_sink_rate input; dt input
% limit the maximum height setpoint from current height depends on maximum
% climb rate, sind rate and dt.
function hgt_sp_adj = fcn(hgt_sp,hgt_sp_prev,max_climb_rate,max_sink_rate,dt)
if ((hgt_sp - hgt_sp_prev) > (max_climb_rate * dt)) 
	hgt_sp_adj = hgt_sp_prev + max_climb_rate * dt;
elseif ((hgt_sp - hgt_sp_prev) < (-max_sink_rate * dt))
	hgt_sp_adj = hgt_sp_prev - max_sink_rate * dt;
else
    hgt_sp_adj = hgt_sp;
	
end

== matlab function V40/FLY_CTRL_SYS/Guidance_Law/TECS/MATLAB Function ==
  data: STE_rate_setpoint input; throttle_predicted output; throttle_cruise input; STE_rate_max input; STE_rate_min input
function throttle_predicted = fcn(STE_rate_setpoint,throttle_cruise,STE_rate_max,STE_rate_min)
if (STE_rate_setpoint >= 0) 
	throttle_predicted = throttle_cruise + STE_rate_setpoint / STE_rate_max * (1.0 - throttle_cruise);

else
    throttle_predicted = throttle_cruise + STE_rate_setpoint / STE_rate_min * (0.0 - throttle_cruise);
end
